simulink model "a2be1"  (R2021a)
settings: Solver=FixedStepAuto  StartTime=0.0  StopTime=100  RelTol=1e-3
settings Model: EnablePacing=on  Creator=Ans Shahzad  LastModifiedBy=Ans Shahzad
settings ConfigComp: DVTestSuiteOptimization=Auto  DVDetectOutOfBounds=on

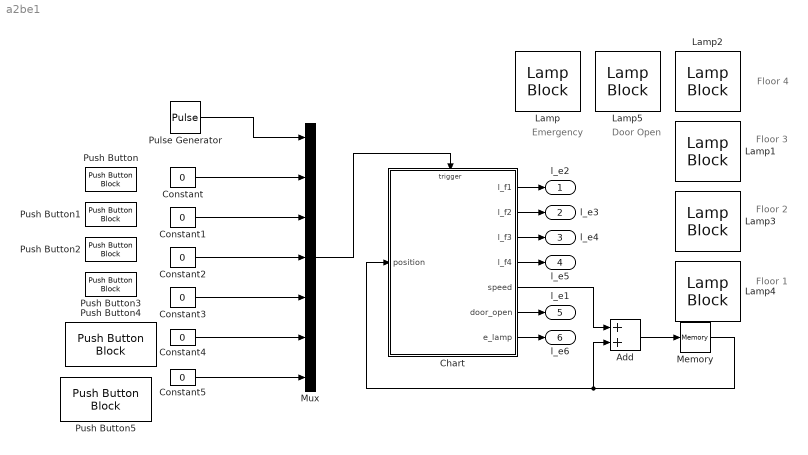
== system a2be1 ==
  note: Floor 1
  note: Floor 2
  note: Floor 3
  note: Floor 4
  note: Door Open
  note: Emergency
  Add : Sum
  Chart : Stateflow chart  TreatAsAtomicUnit=on
  Constant{,1..5} (6 alike) : Constant  Value=0
  Lamp{,1..5} (6 alike) : LampBlock  LabelPosition=Hide
  Memory : Memory  InitialCondition=10
  Mux : Mux  Inputs=7
  Pulse Generator : DiscretePulseGenerator  PulseType=Time based  Period=1  PulseWidth=50
  Push Button : PushButtonBlock  ButtonText=4
  Push Button1 : PushButtonBlock  ButtonText=3
  Push Button2 : PushButtonBlock  ButtonText=2
  Push Button3 : PushButtonBlock  ButtonText=1
  Push Button4 : PushButtonBlock  ButtonText=E
  Push Button5 : PushButtonBlock  ButtonText=S
  l_e2 : Outport
  l_e3 : Outport  Port=2
  l_e4 : Outport  Port=3
  l_e5 : Outport  Port=4
  l_e1 : Outport  Port=5
  l_e6 : Outport  Port=6
  wires:
  Chart/1(l_f1) -> l_e2/1
  Chart/2(l_f2) -> l_e3/1
  Chart/3(l_f3) -> l_e4/1
  Chart/4(l_f4) -> l_e5/1
  Pulse Generator/1 -> Mux/1
  Constant/1 -> Mux/2
  Constant1/1 -> Mux/3
  Constant2/1 -> Mux/4
  Constant3/1 -> Mux/5
  Constant4/1 -> Mux/6
  Constant5/1 -> Mux/7
  Mux/1 -> Chart/Trigger
  Chart/6(door_open) -> l_e1/1
  Add/1 -> Memory/1
  Memory/1 -> Chart/1(position), Add/2
  Chart/7(e_lamp) -> l_e6/1
  Chart/5(speed) -> Add/1

== stateflow chart a2be1/Chart ==
  settings: executeAtInitialization=1
  state Emergency
  state Elevator
    stop = 0;
    on goto_f1: l_f1 = 1;
    queue(f1);
    on goto_f2: l_f2 = 1;
    queue(f2);
    on goto_f3: l_f3 = 1;
    queue(f3);
    on goto_f4: l_f4 = 1;
    queue(f4);
    state Idle
      door_open = false;
      pop;
    state Move
      computeSpeed;
    state Stop
      en:
      lampOff;
      speed = 0;
    (default) -> Idle
    Idle -> Move : [target ~=0]
    Stop -> Idle : [after(5,sec)]
    Move -> Stop : [target == position]{speed = 0; door_open = true;}
  Elevator -> Emergency : Emergency{e_lamp = 1; speed = 0;}
  Emergency -> Elevator : Start{e_lamp = 0;}
  (default) -> Elevator
  data: val function_input; qu local double size=[1 4] =0; l_f1 output; l_f2 output; l_f3 output; l_f4 output; target local; stop local double; speed output; position input; door_open output boolean; e_lamp output; f1 local =10; f3 local =30; f4 local =40; f2 local =20; step local =5
  events: TIC input RISING_EDGE_EVENT; goto_f4 input RISING_EDGE_EVENT; goto_f3 input RISING_EDGE_EVENT; goto_f2 input RISING_EDGE_EVENT; goto_f1 input RISING_EDGE_EVENT; Emergency input RISING_EDGE_EVENT; Start input RISING_EDGE_EVENT
  function queue(val):
    | function queue(val)
    | %        qu(val) = val;
    |         
    |     if (ismember(val,qu) == 0)
    |             i = nnz(qu);
    |             qu(i+1) = val;  
    |     end           
    | end
  function pop:
    | function pop
    |     target = qu(1);
    |     qu(1) = qu(2);
    |     qu(2) = qu(3);
    |     qu(3) = qu(4);
    |     qu(4) = 0;
    |     
    | end
  function computeSpeed:
    | function computeSpeed
    |     if(target > position)
    |         speed = step;
    |     else 
    |         speed = -step;
    |     end
    | end
  function lampOff:
    | function lampOff
    |         switch target
    |             case 10
    |                 l_f1 = f1;
    |             case 20
    |                 l_f2 = f2;
    |             case 30
    |                 l_f3 = f3;
    |             case 40
    |                 l_f4 = f4;
    |         end    
    | end
